simulink model "ficom_pr1_000a_ejemplo_canal_simulinkr14"  (Simulink 4.0)
settings: Solver=ode45  StartTime=0.0  StopTime=20.0  RelTol=1e-3
libraries: commnoisgen2 x3, simulink x2, cstblocks x1
settings Model: Creator=fedemp  LastModifiedBy=fedemp  BooleanDataType=on  RTWOptions="-aEnforceIntegerDowncast=1 -aFoldNonRolledExpr=1 -aInlineInvariantSignals=1 -aInlineParameters=0 -aLocalBlockOutputs=1 -aRollThreshold=5 -aZeroInternalMemoryAtStartup=1 -aZeroExternalMemoryAtStartup=1 -aInitFltsAndDblsToZero=1 -aGenerateReport=0 -aGenCodeOnly=0 -aRTWVerbose=1 -aIncludeHyperlinkInReport=0 -aLaunchReport=0 -aForceParamTrailComments=0 -aGenerateComments=1 -aIgnoreCustomStorageClasses=1 -aIncHierarchyInIds=0 -aMaxRTWIdLen=31 -aShowEliminatedStatements=0 -aPrefixModelToSubsysFcnNames=1 -aIncDataTypeInIds=0 -aInsertBlockDesc=0 -aSimulinkBlockComments=1 -aInlinedPrmAccess=\"Literals\"  -aSuppressErrorStatus=0 -aModelReferenceCompliant=1 -aSupportNonInlinedSFcns=1 -aSupportContinuousTime=1 -aSupportComplex=1 -aSupportNonFinite=1 -aSupportAbsoluteTime=1 -aTargetFcnLib=\"ansi_tfl_tmw.mat\" -aMultiInstanceERTCode=0 -aLogVarNameModifier=\"rt_\" -aIsPILTarget=0 -aCombineOutputUpdateFcns=0 -aGenerateASAP2=0 -aGenerateSampleERTMain=0 -aGenerateFullHeader=1 -aUtilityFuncGeneration=\"Auto\" -aIncludeFileDelimiter=\"Auto\" -aIncludeMdlTerminateFcn=1 -aPurelyIntegerCode=0 -aERTCustomFileBanners=0 -aRTWCAPIStates=0 -aRTWCAPIParams=0 -aRTWCAPISignals=0 -aMatFileLogging=1 -aGenFloatMathFcnCalls=\"ANSI_C\" -aExtModeMexFile=\"ext_comm\" -aExtModeTransport=0 -aExtModeStaticAllocSize=1000000 -aExtModeTesting=0 -aExtModeStaticAlloc=0 -aExtMode=0  -aInitFltsAndDblsToZero=1"

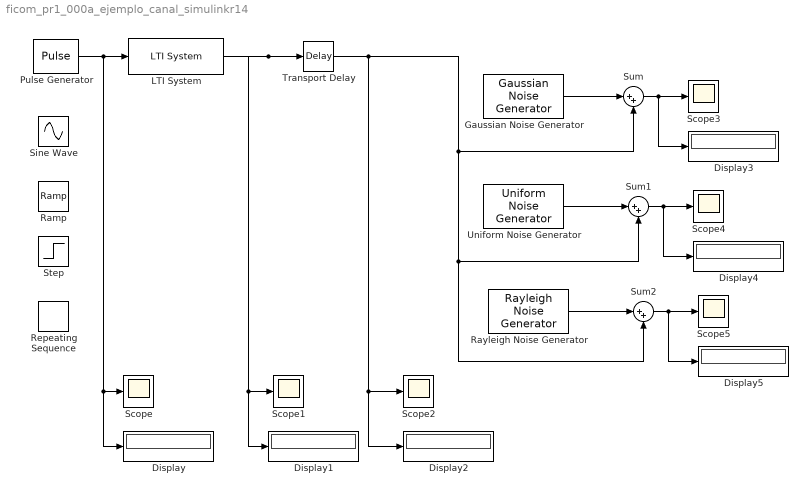
== system ficom_pr1_000a_ejemplo_canal_simulinkr14 ==
  Display{,1..5} (6 alike) : Display
      settings: Format=short
  Gaussian Noise Generator : commnoisgen2/Gaussian Noise Generator  m=0  d=0.6  s=41  Ts=0.01  frameBased=off  sampPerFrame=1  orient=off
  LTI System : cstblocks/LTI System  sys=tf(0.6,[0.5 0.7])  IC=[]
  Pulse Generator : DiscretePulseGenerator  PulseType=Time-based  Amplitude=5  Period=2.5  PulseWidth=40  PhaseDelay=0
  Ramp : simulink/Sources/Ramp  slope=1  start=0  X0=0
  Rayleigh Noise Generator : commnoisgen2/Rayleigh Noise Generator  alpha=1.3  seed=47  Ts=0.01  frameBased=off  sampPerFrame=1  orient=off
  Repeating Sequence : simulink/Sources/Repeating Sequence  rep_seq_t=[0 2]  rep_seq_y=[0 2]
  Scope{,1..5} (6 alike) : Scope
      Scope settings: TimeRange=auto  YMin=-5  YMax=5  SaveToWorkspace=off  SaveName=ScopeData  LimitDataPoints=on  MaxDataPoints=5000
      Scope1 settings: TimeRange=auto  YMin=-5  YMax=5  SaveToWorkspace=off  LimitDataPoints=on  MaxDataPoints=5000
      Scope2 settings: TimeRange=auto  YMin=-5  YMax=5  SaveToWorkspace=off  SaveName=ScopeData2  LimitDataPoints=on  MaxDataPoints=5000
      Scope3 settings: TimeRange=auto  YMin=-5  YMax=5  SaveToWorkspace=off  SaveName=ScopeData3  LimitDataPoints=on  MaxDataPoints=5000
      Scope4 settings: TimeRange=auto  YMin=-5  YMax=5  SaveToWorkspace=off  SaveName=ScopeData4  LimitDataPoints=on  MaxDataPoints=5000
      Scope5 settings: TimeRange=auto  YMin=-5  YMax=5  SaveToWorkspace=off  SaveName=ScopeData5  LimitDataPoints=on  MaxDataPoints=5000
  Sine Wave : Sin  SineType=Time-based  Amplitude=5  Bias=0  Frequency=0.6  Phase=0.6  Samples=10  Offset=0
  Step : Step  Time=1  Before=0  After=1
  Sum : Sum  Inputs=|++  SaturateOnIntegerOverflow=off
  Sum1 : Sum  Inputs=|++  SaturateOnIntegerOverflow=off
  Sum2 : Sum  Inputs=|++  SaturateOnIntegerOverflow=off
  Transport Delay : TransportDelay  DelayTime=0.6  InitialInput=0  BufferSize=1024  PadeOrder=0
  Uniform Noise Generator : commnoisgen2/Uniform Noise Generator  low=0  up=1  seed=31  Ts=0.01  frameBased=off  sampPerFrame=1  orient=off
  wires:
  Pulse Generator/1 -> LTI System/1, Scope/1, Display/1
  LTI System/1 -> Transport Delay/1, Scope1/1, Display1/1
  Transport Delay/1 -> Sum/2, Sum1/2, Sum2/2, Scope2/1, Display2/1
  Gaussian Noise Generator/1 -> Sum/1
  Sum/1 -> Scope3/1, Display3/1
  Uniform Noise Generator/1 -> Sum1/1
  Sum1/1 -> Scope4/1, Display4/1
  Rayleigh Noise Generator/1 -> Sum2/1
  Sum2/1 -> Scope5/1, Display5/1
